simulink model "simple_test_jitter"  (Simulink 7.8)
settings: Solver=VariableStepDiscrete  StartTime=0.0  StopTime=10^-3  RelTol=1e-3
settings Model: Creator=chuh  LastModifiedBy=chuh

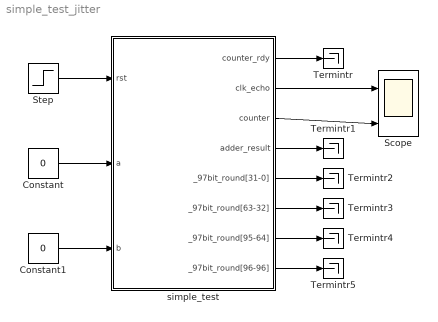
== system simple_test_jitter ==
  Constant : Constant  Value=0
  Constant1 : Constant  Value=0
  Scope : Scope  NumInputPorts=2
      settings: YMin=-5~0  YMax=5~1000  SaveName=sim_result  SampleInput=on  SampleTime=10^-9
  Step : Step  Time=(10^-9)*2  Before=1  After=0  SampleTime=0
  Termintr{,1..5} (6 alike) : Terminator
  simple_test : Subsystem  mask(simple_test){params_samples=1e-09, params_freq=1}
      mask prompts: params_samples "Sample time:"; params_freq "FPGA frequency (MHz):"
      mask help:
      | input rst
      | input a[30:0]
      | input b[30:0]
      | output counter_rdy
      | output clk_echo
      | output counter[15:0]
      | output adder_result[31:0]
      | output _97bit_round[96:0]
      mask Help:
      | input rst
      | input a[30:0]
      | input b[30:0]
      | output counter_rdy
      | output clk_echo
      | output counter[15:0]
      | output adder_result[31:0]
      | output _97bit_round[96:0]
  wires:
  Step/1 -> simple_test/1(rst)
  Constant/1 -> simple_test/2(a)
  Constant1/1 -> simple_test/3(b)
  simple_test/2(clk_echo) -> Scope/1
  simple_test/3(counter) -> Scope/2
  simple_test/1(counter_rdy) -> Termintr/1
  simple_test/4(adder_result) -> Termintr1/1
  simple_test/5(_97bit_round[31-0]) -> Termintr2/1
  simple_test/6(_97bit_round[63-32]) -> Termintr3/1
  simple_test/7(_97bit_round[95-64]) -> Termintr4/1
  simple_test/8(_97bit_round[96-96]) -> Termintr5/1

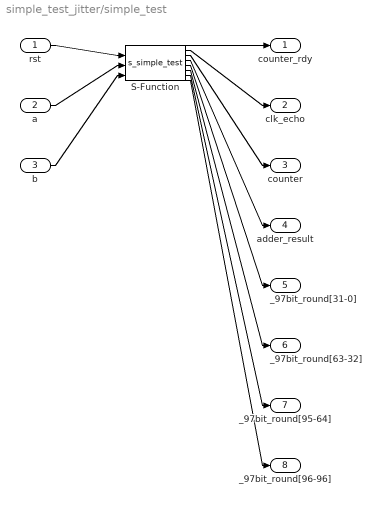
== system simple_test_jitter/simple_test ==
  rst : Inport  OutDataTypeStr=double  SampleTime=1e-09
  a : Inport  Port=2  OutDataTypeStr=double  SampleTime=1e-09
  b : Inport  Port=3  OutDataTypeStr=double  SampleTime=1e-09
  S-Function : S-Function  FunctionName=s_simple_test  Parameters=params_samples, params_freq  EnableBusSupport=off
  counter_rdy : Outport  OutDataTypeStr=uint32  SampleTime=1e-09
  clk_echo : Outport  Port=2  OutDataTypeStr=uint32  SampleTime=1e-09
  counter : Outport  Port=3  OutDataTypeStr=uint32  SampleTime=1e-09
  adder_result : Outport  Port=4  OutDataTypeStr=uint32  SampleTime=1e-09
  _97bit_round[31-0] : Outport  Port=5  OutDataTypeStr=uint32  SampleTime=1e-09
  _97bit_round[63-32] : Outport  Port=6  OutDataTypeStr=uint32  SampleTime=1e-09
  _97bit_round[95-64] : Outport  Port=7  OutDataTypeStr=uint32  SampleTime=1e-09
  _97bit_round[96-96] : Outport  Port=8  OutDataTypeStr=uint32  SampleTime=1e-09
  wires:
  rst/1 -> S-Function/1
  a/1 -> S-Function/2
  b/1 -> S-Function/3
  S-Function/1 -> counter_rdy/1
  S-Function/2 -> clk_echo/1
  S-Function/3 -> counter/1
  S-Function/4 -> adder_result/1
  S-Function/5 -> _97bit_round[31-0]/1
  S-Function/6 -> _97bit_round[63-32]/1
  S-Function/7 -> _97bit_round[95-64]/1
  S-Function/8 -> _97bit_round[96-96]/1
